simulink subsystem "MotorInteraction"  (R2024b)
settings: Solver=VariableStepAuto  StartTime=0.0  StopTime=10.0  RelTol=1e-3
model mask{whangle=0}
  mask prompts: whangle "Wheel angle [rad]"
undefined symbols (not defined in the file): motor, wheels
settings Model: Creator=Marij  LastModifiedBy=marijn

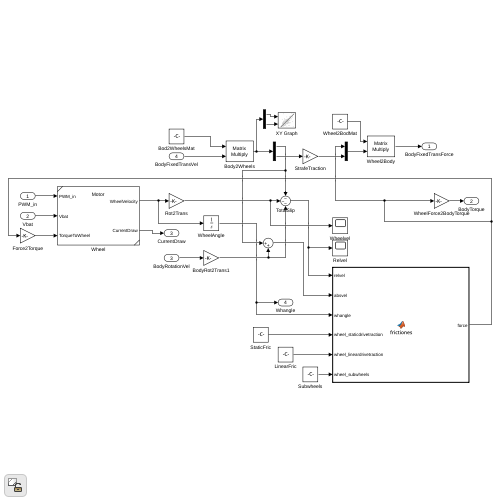
[thumbnail: Simulink's stored preview of the top-level diagram]
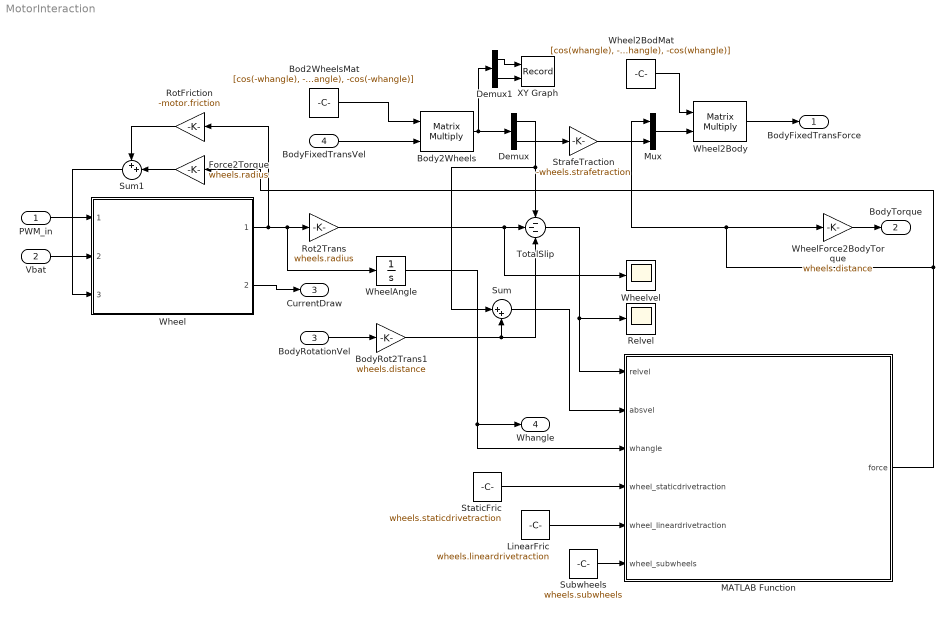
== system MotorInteraction ==
  PWM_in : Inport
  Vbat : Inport  Port=2
  BodyRotationVel : Inport  Port=3  Unit=rad/s
  BodyFixedTransVel : Inport  Port=4  Unit=m/s  PortDimensions=2
  Bod2WheelsMat : Constant  Value=[cos(-whangle), -sin(-whangle); sin(-whangle), -cos(-whangle)]  VectorParams1D=off
  Body2Wheels : Product  Multiplication=Matrix(*)
  BodyRot2Trans1 : Gain  Gain=wheels.distance
  Demux : Demux  Outputs=2
  Demux1 : Demux  Outputs=2
  Force2Torque : Gain  Gain=wheels.radius
  LinearFric : Constant  Value=wheels.lineardrivetraction
  MATLAB Function : MATLAB Function  TreatAsAtomicUnit=on
  Mux : Mux  Inputs=2
  Relvel : Scope
  Rot2Trans : Gain  Gain=wheels.radius
  RotFriction : Gain  Gain=-motor.friction
  StaticFric : Constant  Value=wheels.staticdrivetraction
  StrafeTraction : Gain  Gain=-wheels.strafetraction
  Subwheels : Constant  Value=wheels.subwheels
  Sum : Sum  Inputs=|++
  Sum1 : Sum  Inputs=++|
  TotalSlip : Sum  Inputs=---
  Wheel : Subsystem  ReferencedSubsystem=Motor
  Wheel2BodMat : Constant  Value=[cos(whangle), -sin(whangle); sin(whangle), -cos(whangle)]  VectorParams1D=off
  Wheel2Body : Product  Multiplication=Matrix(*)
  WheelAngle : Integrator
  WheelForce2BodyTorque : Gain  Gain=wheels.distance
  Wheelvel : Scope
  XY Graph : Record  FileSettingsInternal="{\"entries\":[{\"content\":{\"excelSettings\":{\"content\":{},\"type\":\"Streamout.ExcelSettings\"}},\"type\":\"Streamout.FileSettingStorage\",\"uuid\":\"\"}],\"packageUris\":[\"http:\\/\\/schema.mathworks.com\\/mf0\\/streamout_blocks\\/R2020a\"],\"version\":\"1.0\"}"  Layout=[1 1]  SignalsInternal="{\"entries\":[{\"content\":{\"signals\":[{\"content\":{\"blockPath\":[],\"dimensions\":[1],\"domain\":\"\",\"lineColor\":\"#a2142f\",\"plots\":[ 1 ],\"port\":1,\"signalID\":1,\"signalName\":\"XY Graph:1\"},\"type\":\"RecordBlkView.Signal\",\"uuid\":\"\"},{\"content\":{\"blockPath\":[],\"dimensions\":[1],\"domain\":\"\",\"lineColor\":\"#139fff\",\"plots\":[ 1 ],\"port\":2,\"signalID\":2,\"signalName\":\"XY Graph:2\"},\"type\":\"RecordBlkView.Signal\",\"uuid\":\"\"}]},\"type\":\"RecordBlkView.InputSignals\",\"uuid\":\"\"}],\"packageUris\":[\"http:\\/\\/schema.mathworks.com\\/mf0\\/streamout_blocks\\/R2020a\"],\"version\":\"1.0\"}"  VisualizationBindings="{\"xyplotplugin\":{\"info\":[{\"series\":[{\"bindingParametersList\":[{\"parameter\":\"X-Axis\",\"signalID\":1,\"signalName\":\"XY Graph:1\"},{\"parameter\":\"Y-Axis\",\"signalID\":2,\"signalName\":\"XY Graph:2\"}],\"seriesID\":0}],\"subplotID\":1}]}}"  CompatibilityTag=XY
  BodyFixedTransForce : Outport  Unit=N  PortDimensions=2
  BodyTorque : Outport  Port=2  Unit=N*m
  CurrentDraw : Outport  Port=3  Unit=A  PortDimensions=1
  Whangle : Outport  Port=4
  wires:
  WheelForce2BodyTorque/1 -> BodyTorque/1
  BodyRotationVel/1 -> BodyRot2Trans1/1
  Body2Wheels/1 -> Demux1/1, Demux/1
  StaticFric/1 -> MATLAB Function/4(wheel_staticdrivetraction)
  Demux/1 -> Sum/1, TotalSlip/1
  Subwheels/1 -> MATLAB Function/6(wheel_subwheels)
  Wheel2Body/1 -> BodyFixedTransForce/1
  LinearFric/1 -> MATLAB Function/5(wheel_lineardrivetraction)
  MATLAB Function/1(force) -> Force2Torque/1, WheelForce2BodyTorque/1, Mux/1
  Demux/2 -> StrafeTraction/1
  BodyRot2Trans1/1 -> Sum/2, TotalSlip/3
  Wheel2BodMat/1 -> Wheel2Body/1
  TotalSlip/1 -> Relvel/1, MATLAB Function/1(relvel)
  StrafeTraction/1 -> Mux/2
  Wheel/2 -> CurrentDraw/1
  Mux/1 -> Wheel2Body/2
  Sum/1 -> MATLAB Function/2(absvel)
  PWM_in/1 -> Wheel/1
  Wheel/1 -> RotFriction/1, WheelAngle/1, Rot2Trans/1
  WheelAngle/1 -> Whangle/1, MATLAB Function/3(whangle)
  Rot2Trans/1 -> Wheelvel/1, TotalSlip/2
  Vbat/1 -> Wheel/2
  BodyFixedTransVel/1 -> Body2Wheels/2
  Bod2WheelsMat/1 -> Body2Wheels/1
  Demux1/2 -> XY Graph/2
  Demux1/1 -> XY Graph/1
  Force2Torque/1 -> Sum1/2
  RotFriction/1 -> Sum1/1
  Sum1/1 -> Wheel/3

== matlab function MotorInteraction/MATLAB Function ==
  data: relvel input; force output; absvel input; whangle input; wheel_staticdrivetraction input; wheel_lineardrivetraction input; wheel_subwheels input
function force = frictiones(relvel, absvel, whangle, wheel_staticdrivetraction, wheel_lineardrivetraction, wheel_subwheels)
force = drivetraction_model(relvel, absvel, whangle, wheel_staticdrivetraction, wheel_lineardrivetraction, wheel_subwheels);
% force = drivetraction_linear(relvel, absvel, whangle, wheel_staticdrivetraction, wheel_lineardrivetraction, wheel_subwheels);
end
